simulink model "Sudarshan_1_lab_6"  (R2022b)
settings: Solver=VariableStepAuto  StartTime=0.0  StopTime=10.0  RelTol=1e-3
settings Model: Creator=year2  LastModifiedBy=year2

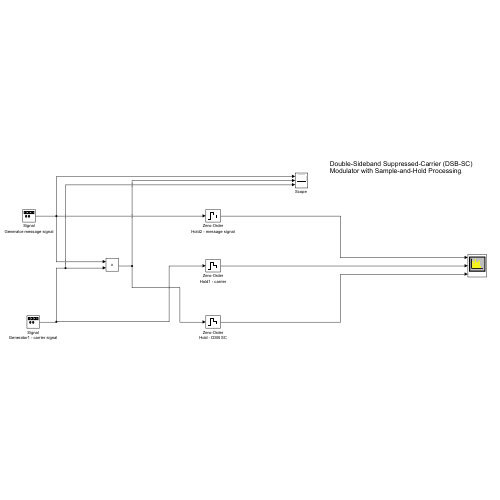
[thumbnail: Simulink's stored preview of the top-level diagram]
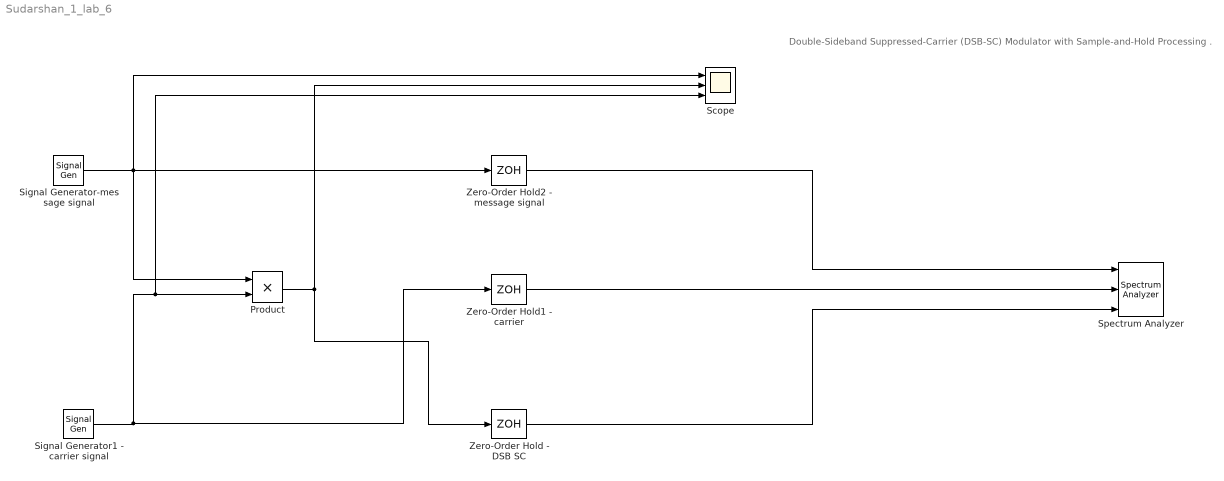
== system Sudarshan_1_lab_6 ==
  note: Double-Sideband Suppressed-Carrier (DSB-SC) Modulator with Sample-and-Hold Processing .
  Product : Product
  "Scope " : Scope  NumInputPorts=3
  Signal Generator-message signal : SignalGenerator  Frequency=200
  Signal Generator1 - carrier signal : SignalGenerator  Frequency=1500
  Spectrum Analyzer : SpectrumAnalyzer  NumInputPorts=3
  Zero-Order Hold - DSB SC : ZeroOrderHold  SampleTime=-1
  Zero-Order Hold1 - carrier : ZeroOrderHold  SampleTime=-1
  Zero-Order Hold2 - message signal : ZeroOrderHold  SampleTime=-1
  wires:
  Signal Generator-message signal/1 -> "Scope "/1, Zero-Order Hold2 - message signal/1, Product/1
  Signal Generator1 - carrier signal/1 -> Zero-Order Hold1 - carrier/1, "Scope "/3, Product/2
  Product/1 -> "Scope "/2, Zero-Order Hold - DSB SC/1
  Zero-Order Hold2 - message signal/1 -> Spectrum Analyzer/1
  Zero-Order Hold1 - carrier/1 -> Spectrum Analyzer/2
  Zero-Order Hold - DSB SC/1 -> Spectrum Analyzer/3
